simulink model "pro3"  (R2020a)
settings: Solver=VariableStepAuto  StartTime=0.0  StopTime=10.0  RelTol=1e-3
settings Model: Creator=aa  LastModifiedBy=aa

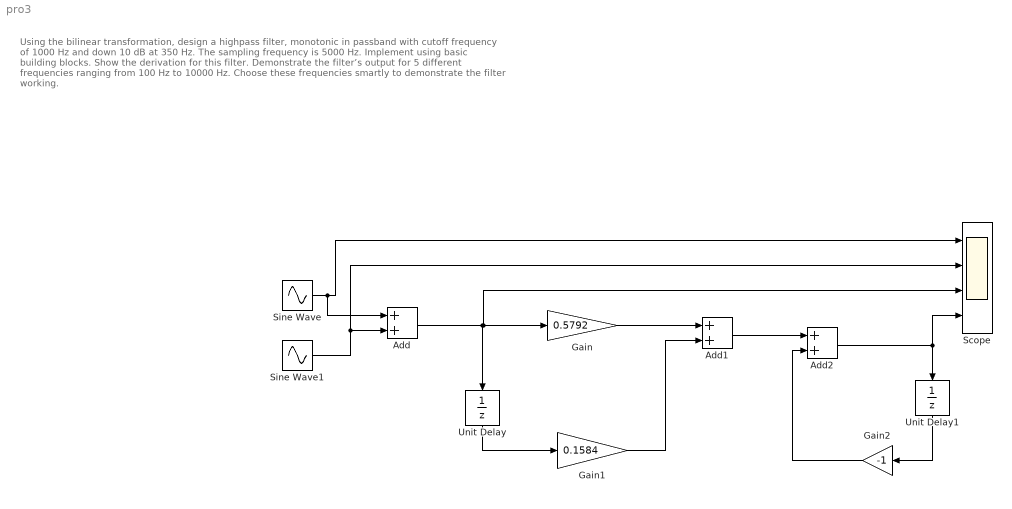
== system pro3 ==
  note: Using the bilinear transformation, design a highpass filter, monotonic in passband with cutoff frequency of 1000 Hz and down 10 dB at 350 Hz. The sampling frequency is 5000 Hz. Implement using basic building blocks. Show the derivation for this filter. Demonstrate the filter’s output for 5 different frequencies ranging from 100 Hz to 10000 Hz. Choose these frequencies smartly to demonstrate the filter working.
  Add : Sum
  Add1 : Sum
  Add2 : Sum
  Gain : Gain  Gain=0.5792
  Gain1 : Gain  Gain=0.1584
  Gain2 : Gain  Gain=-1
  Scope : Scope  NumInputPorts=4
  Sine Wave : Sin  SampleTime=0
  Sine Wave1 : Sin  Frequency=200  SampleTime=0
  Unit Delay : UnitDelay  SampleTime=-1  HasFrameUpgradeWarning=on
  Unit Delay1 : UnitDelay  SampleTime=-1  HasFrameUpgradeWarning=on
  wires:
  Gain1/1 -> Add1/2
  Sine Wave1/1 -> Scope/2, Add/2
  Add/1 -> Unit Delay/1, Scope/3, Gain/1
  Sine Wave/1 -> Add/1, Scope/1
  Add1/1 -> Add2/1
  Add2/1 -> Unit Delay1/1, Scope/4
  Gain2/1 -> Add2/2
  Unit Delay/1 -> Gain1/1
  Unit Delay1/1 -> Gain2/1
  Gain/1 -> Add1/1
